simulink model "simulink_model_pid_controller_IT2"  (R2022b)
settings: Solver=ode1be  StartTime=0.0  StopTime=10  RelTol=1e-3
libraries: slpidlib x1
settings Model: Creator=giris  LastModifiedBy=giris

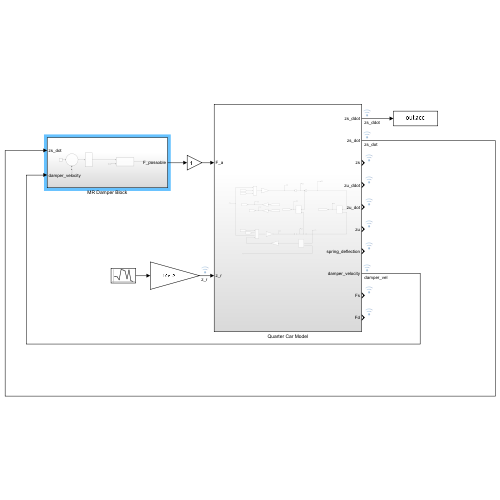
[thumbnail: Simulink's stored preview of the top-level diagram]
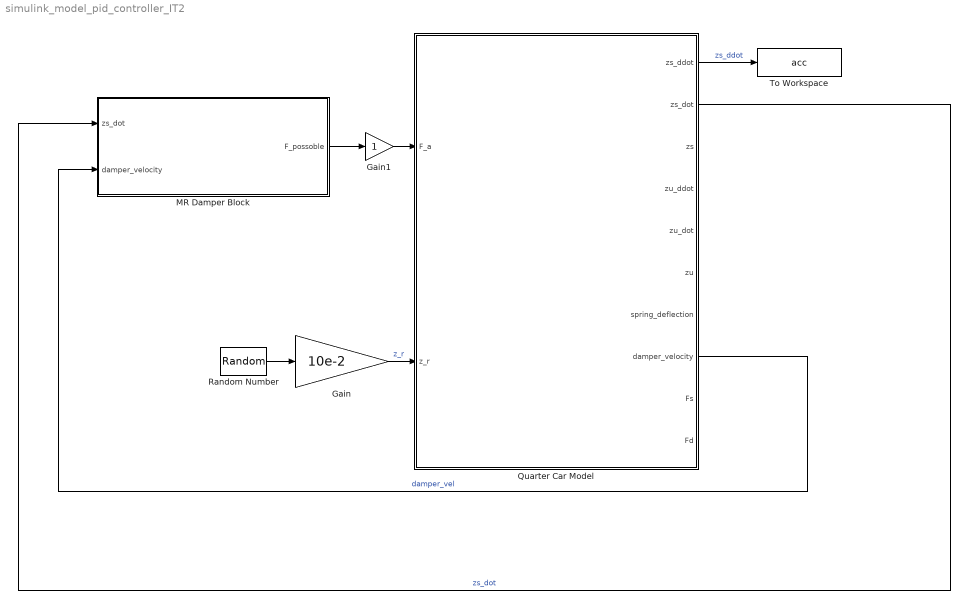
== system simulink_model_pid_controller_IT2 ==
  Gain : Gain  Gain=10e-2
  Gain1 : Gain
  MR Damper Block : Subsystem
  Quarter Car Model : Subsystem
  Random Number : RandomNumber  SampleTime=0.01
  To Workspace : ToWorkspace  VariableName=acc  SaveFormat=Timeseries  SampleTime=-1
  wires:
  Random Number/1 -> Gain/1
  Gain/1 -> Quarter Car Model/2(z_r)  "z_r"
  Quarter Car Model/8(damper_velocity) -> MR Damper Block/2(damper_velocity)  "damper_vel"
  Quarter Car Model/2(zs_dot) -> MR Damper Block/1(zs_dot)  "zs_dot"
  Quarter Car Model/1(zs_ddot) -> To Workspace/1  "zs_ddot"
  MR Damper Block/1(F_possoble) -> Gain1/1
  Gain1/1 -> Quarter Car Model/1(F_a)

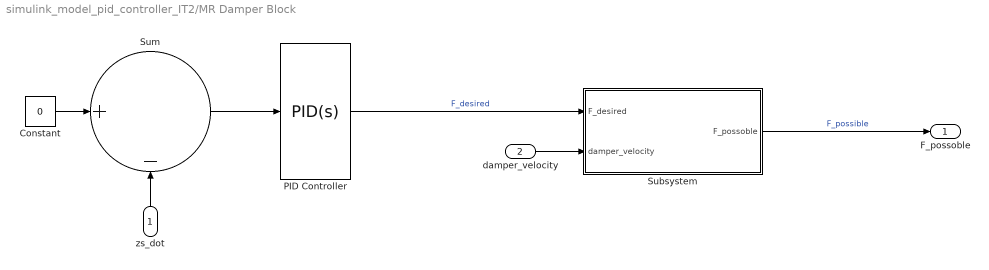
== system simulink_model_pid_controller_IT2/MR Damper Block ==
  zs_dot : Inport
  damper_velocity : Inport  Port=2
  Constant : Constant  Value=0
  PID Controller : slpidlib/PID Controller  Controller=PID  Form=Parallel  TimeDomain=Continuous-time  UseExternalTs=off  SampleTime=-1  IntegratorMethod=Forward Euler  FilterMethod=Forward Euler  ControllerParametersSource=internal  P=4000  I=500  UseKiTs=off  D=800  N=2000  UseFilter=on  TunerSelectOption=Transfer Function Based (PID Tuner App)  InitialConditionSource=internal  InitialConditionForIntegrator=0  InitialConditionForFilter=0  DifferentiatorICPrevScaledInput=0  ExternalReset=none  TrackingMode=off  Kt=1  LimitOutput=off  SatLimitsSource=internal  UpperSaturationLimit=inf  LowerSaturationLimit=-inf  LinearizeAsGain=on  AntiWindupMode=none  Kb=1  LimitIntegrator=off  UpperIntegratorSaturationLimit=inf  LowerIntegratorSaturationLimit=-inf  POutMin=[]  POutMax=[]  IOutMin=[]  IOutMax=[]  DOutMin=[]  DOutMax=[]  NOutMin=[]  NOutMax=[]  SumOutMin=[]  SumOutMax=[]  SaturationOutMin=[]  SaturationOutMax=[]  PParamMin=[]  PParamMax=[]  IParamMin=[]  IParamMax=[]  DParamMin=[]  DParamMax=[]  NParamMin=[]  NParamMax=[]  KbParamMin=[]  KbParamMax=[]  KtParamMin=[]  KtParamMax=[]  KbOutMin=[]  KbOutMax=[]  KtOutMin=[]  KtOutMax=[]  IntegratorOutMin=[]  IntegratorOutMax=[]  FilterOutMin=[]  FilterOutMax=[]  SumI1OutMin=[]  SumI1OutMax=[]  SumI2OutMin=[]  SumI2OutMax=[]  SumI3OutMin=[]  SumI3OutMax=[]  SumI4OutMin=[]  SumI4OutMax=[]  SumDOutMin=[]  SumDOutMax=[]  DifferentiatorOutMin=[]  DifferentiatorOutMax=[]  FilterDiffOutCoefMin=[]  FilterDiffOutCoefMax=[]  ReciprocalOutMin=[]  ReciprocalOutMax=[]  SumDenOutMin=[]  SumDenOutMax=[]  SumNumOutMin=[]  SumNumOutMax=[]  DivideOutMin=[]  DivideOutMax=[]  UdiffTsProdOutMin=[]  UdiffTsProdOutMax=[]  NTsProdOutMin=[]  NTsProdOutMax=[]  UintegralTsProdOutMin=[]  UintegralTsProdOutMax=[]  UngainTsProdOutMin=[]  UngainTsProdOutMax=[]  ClampingZeroOutDataTypeStr=Inherit: Inherit via back propagation  ClampingZeroOutMin=[]  ClampingZeroOutMax=[]  FilterDenConstantOutDataTypeStr=Inherit: Inherit via back propagation  FilterDenConstantOutMin=[]  FilterDenConstantOutMax=[]  PCopyOutDataTypeStr=Inherit: Inherit via back propagation  PCopyOutMin=[]  PCopyOutMax=[]  NCopyOutDataTypeStr=Inherit: Inherit via back propagation  NCopyOutMin=[]  NCopyOutMax=[]  IntegratorContinuousStateAttributes=''  IntegratorStateMustResolveToSignalObject=off  IntegratorRTWStateStorageClass=Auto  FilterContinuousStateAttributes=''  FilterStateMustResolveToSignalObject=off  FilterRTWStateStorageClass=Auto  ParallelPVariant=InternalParameters  IdealPVariant=Disabled  IVariant=InternalParameters  DVariant=InternalParameters  IntegratorVariant=Continuous  SatVariant=Disabled  AWVariant=Passthrough  PCopyVariant=Disabled  TRVariant=Disabled  FdbkBlocksVariant=Forward  IdealPFdbkVariant=Disabled  SatFdbkVariant=Disabled  DerivativeFilterVariant=ContFilter  NVariant=InternalParameters  NCopyVariant=Disabled  FilterICVariant=InternalICsFilter  IntegratorICVariant=InternalICs  ExternalResetVariant=Disabled  TRSumVariant=Passthrough  SumFdbkVariant=Disabled  SumVariant=Sum_PID  TsampFilterVariant=InternalTs  TsampNgainVariant=Passthrough  TsampIntegralVariant=Passthrough  ExternalSaturationOutDataTypeStr=Inherit: Same as second input
  Subsystem : Subsystem
  Sum : Sum  Inputs=|+-
  F_possoble : Outport
  wires:
  PID Controller/1 -> Subsystem/1(F_desired)  "F_desired"
  Subsystem/1(F_possoble) -> F_possoble/1  "F_possible"
  Sum/1 -> PID Controller/1
  Constant/1 -> Sum/1
  zs_dot/1 -> Sum/2
  damper_velocity/1 -> Subsystem/2(damper_velocity)

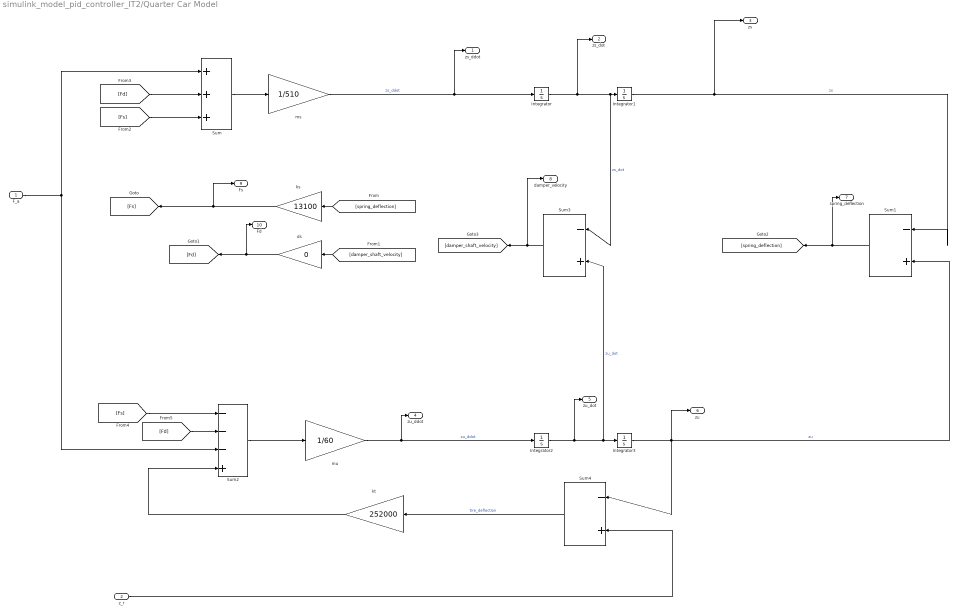
== system simulink_model_pid_controller_IT2/Quarter Car Model ==
  F_a : Inport
  z_r : Inport  Port=2
  Integrator{,1..3} (4 alike) : Integrator
  Sum : Sum  Inputs=+++
  Sum1 : Sum  Inputs=|-+
  Sum2 : Sum  Inputs=---+
  Sum3 : Sum  Inputs=|-+
  Sum4 : Sum  Inputs=|-+
  ds : Gain  Gain=0
  ks : Gain  Gain=13100
  kt : Gain  Gain=252000
  ms : Gain  Gain=1/510
  mu : Gain  Gain=1/60
  zs_ddot : Outport
  zs_dot : Outport  Port=2
  zs : Outport  Port=3
  zu_ddot : Outport  Port=4
  zu_dot : Outport  Port=5
  zu : Outport  Port=6
  spring_deflection : Outport  Port=7
  damper_velocity : Outport  Port=8
  Fs : Outport  Port=9
  Fd : Outport  Port=10
  wires:
  [spring_deflection] -> ks/1
  [damper_shaft_velocity] -> ds/1
  Integrator/1 -> zs_dot/1, Sum3/1, Integrator1/1  "zs_dot"
  Integrator1/1 -> zs/1, Sum1/1  "zs"
  Sum/1 -> ms/1
  [Fs] -> Sum/3
  ks/1 -> Fs/1, [Fs]
  ds/1 -> Fd/1, [Fd]
  [Fd] -> Sum/2
  F_a/1 -> Sum/1, Sum2/3
  Sum1/1 -> spring_deflection/1, [spring_deflection]
  [Fs] -> Sum2/1
  [Fd] -> Sum2/2
  Sum2/1 -> mu/1
  Integrator2/1 -> zu_dot/1, Sum3/2, Integrator3/1  "zu_dot"
  Integrator3/1 -> Sum4/1, Sum1/2, zu/1  "zu"
  Sum3/1 -> damper_velocity/1, [damper_shaft_velocity]
  kt/1 -> Sum2/4
  Sum4/1 -> kt/1  "tire_deflection"
  z_r/1 -> Sum4/2
  ms/1 -> zs_ddot/1, Integrator/1  "zs_ddot"
  mu/1 -> zu_ddot/1, Integrator2/1  "zu_ddot"

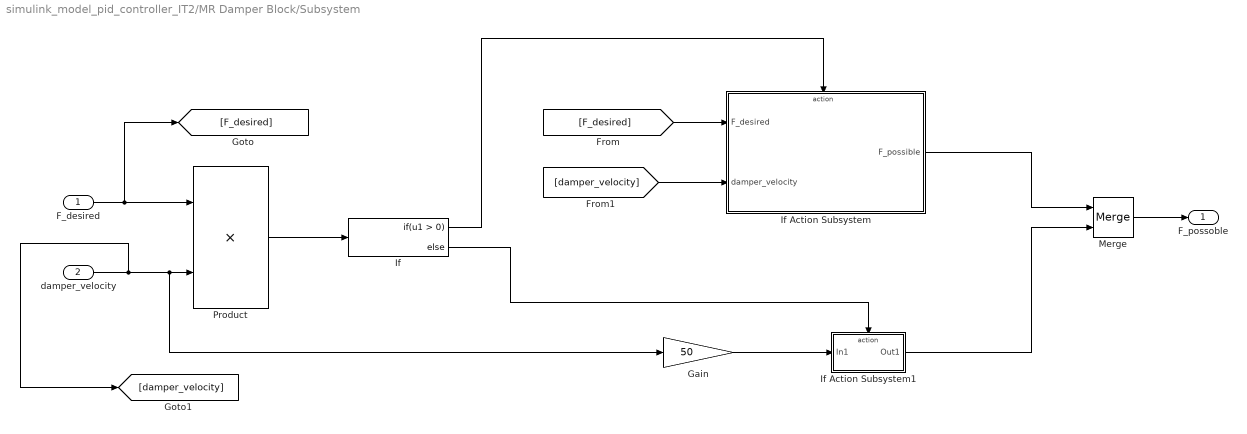
== system simulink_model_pid_controller_IT2/MR Damper Block/Subsystem ==
  F_desired : Inport
  damper_velocity : Inport  Port=2
  Gain : Gain  Gain=50
  If : If
  If Action Subsystem : Subsystem  TreatAsAtomicUnit=on
  If Action Subsystem1 : Subsystem  TreatAsAtomicUnit=on
  Merge : Merge
  Product : Product
  F_possoble : Outport
  wires:
  F_desired/1 -> [F_desired], Product/1
  damper_velocity/1 -> [damper_velocity], Gain/1, Product/2
  Product/1 -> If/1
  If/1 -> If Action Subsystem/Action
  If Action Subsystem/1(F_possible) -> Merge/1
  Merge/1 -> F_possoble/1
  If/2 -> If Action Subsystem1/Action
  Gain/1 -> If Action Subsystem1/1(In1)
  If Action Subsystem1/1(Out1) -> Merge/2
  [F_desired] -> If Action Subsystem/1(F_desired)
  [damper_velocity] -> If Action Subsystem/2(damper_velocity)

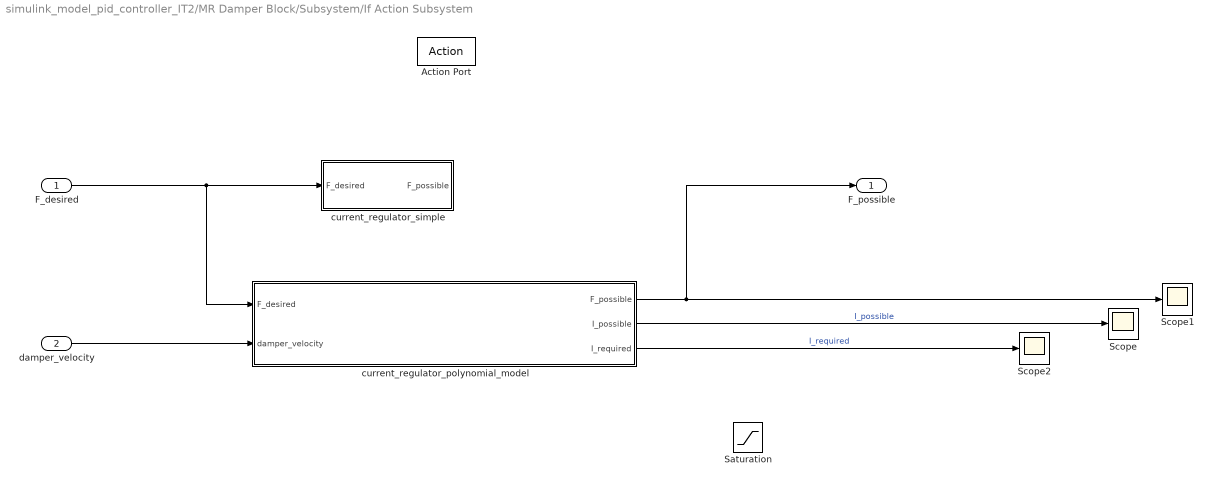
== system simulink_model_pid_controller_IT2/MR Damper Block/Subsystem/If Action Subsystem ==
  F_desired : Inport
  damper_velocity : Inport  Port=2
  Action Port : ActionPort  ActionPortLabel=if(u1 > 0)
  Saturation : Saturate  UpperLimit=2000  LowerLimit=-2000
  Scope : Scope
  Scope1 : Scope
  Scope2 : Scope
  current_regulator_polynomial_model : MATLAB Function  TreatAsAtomicUnit=on
  current_regulator_simple : MATLAB Function  TreatAsAtomicUnit=on
  F_possible : Outport
  wires:
  damper_velocity/1 -> current_regulator_polynomial_model/2(damper_velocity)
  F_desired/1 -> current_regulator_polynomial_model/1(F_desired), current_regulator_simple/1(F_desired)
  current_regulator_polynomial_model/1(F_possible) -> F_possible/1, Scope1/1
  current_regulator_polynomial_model/2(I_possible) -> Scope/1  "I_possible"
  current_regulator_polynomial_model/3(I_required) -> Scope2/1  "I_required"

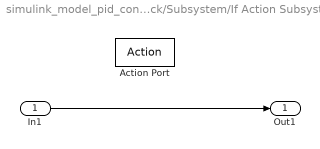
== system simulink_model_pid_controller_IT2/MR Damper Block/Subsystem/If Action Subsystem1 ==
  In1 : Inport
  Action Port : ActionPort  ActionPortLabel=else
  Out1 : Outport
  wires:
  In1/1 -> Out1/1

== matlab function simulink_model_pid_controller_IT2/MR Damper Block/Subsystem/If Action Subsystem/current_regulator_polynomial_model ==
  data: F_desired input; F_possible output; damper_velocity input; I_possible output; I_required output
function [F_possible, I_possible, I_required] = current_regulator_polynomial_model(F_desired, damper_velocity)


v = damper_velocity*1;
I_max = 0.5;

c0 = -659.4;
c1 = 8.995;
c2 = 0.1062;
c3 = -1.584e-4;
c4 = -5.908e-6;
c5 = 1.137e-9;
c6 = 1.087e-10;
c7 = 0;
c8 = 0;
c9 = 0;
c10 = 0;
c11 = 0;


I_required = (F_desired)/(1000*(0*c0*v^0 + c1*v^1 + c2*v^2 + c3*v^3 + c4*v^4 + c5*v^5 + c6*v^6 + c7*v^7 + c8*v^8 + c9*v^9 + c10*v^10 + c11*v^11));

if abs(I_required) > I_max
    I_possible = I_max;
else
    I_possible = I_required;
end


F_possible = (1000*(0*c0*v^0 + c1*v^1 + c2*v^2 + c3*v^3 + c4*v^4 + c5*v^5 + c6*v^6 + c7*v^7 + c8*v^8 + c9*v^9 + c10*v^10 + c11*v^11))*I_possible;

== matlab function simulink_model_pid_controller_IT2/MR Damper Block/Subsystem/If Action Subsystem/current_regulator_simple ==
  data: F_desired input; F_possible output
function F_possible = current_regulator_simple(F_desired)

cs = 1000; % N/A

I_required = F_desired/cs;

I_max = 3;

if abs(I_required) > I_max

    I_possible = sign(F_desired)*I_max;

else

    I_possible = I_required;

end

F_possible = I_possible * cs;
